simulink model "optimizer"  (R2020a)
settings: Solver=VariableStepAuto  StartTime=0.0  StopTime=10.0  RelTol=1e-3
settings Model: Creator=PIM  LastModifiedBy=PIM

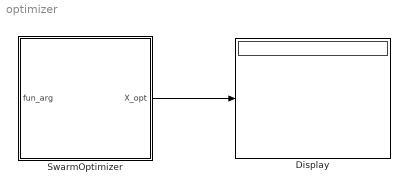
== system optimizer ==
  Display : Display
  SwarmOptimizer : MATLAB Function  TreatAsAtomicUnit=on  mask{algorithm_mask=Differential Evolution Optimizer, n_iter=100, n_particles=50, sampling_method_mask=Uniform, domain_hi=[5 5 5], domain_lo=[-5 -5 -5]}
      mask prompts: algorithm_mask "Algorithm"; n_iter "Number of iterations [float]"; n_particles "Number of particles [float]"; sampling_method_mask "Sampling method"; domain_hi "Domain Hi (array) [float]"; domain_lo "Domain Lo (array) [float]"
      mask init:
      | if strcmp(sampling_method_mask, 'Uniform')
      |     sampling_method=1;
      | elseif strcmp(sampling_method_mask, 'Cauchy')
      |     sampling_method=2;
      | elseif strcmp(sampling_method_mask, 'Normal')
      |     sampling_method=3;
      | end
      | 
      | if strcmp(algorithm_mask, 'Particle Swarm Optimizer')
      |     algorithm=1;
      | elseif strcmp(algorithm_mask, 'Differential Evolution Optimizer')
      |     algorithm=2;
      | end
  wires:
  SwarmOptimizer/1(X_opt) -> Display/1

== matlab function optimizer/SwarmOptimizer ==
  data: fun_arg input; n_particles parameter double; n_iter parameter double; domain_hi parameter double; domain_lo parameter double; sampling_method parameter double; algorithm parameter double; X_opt output size=size(domain_hi)
function X_opt=fcn(fun_arg, n_particles, n_iter, domain_hi, domain_lo, sampling_method, algorithm)
% global swarm_obj
% global topology_obj

swarm_obj=swarm;
topology_obj=topology;

%% Swarm parameters
swarm_param.n_particles=n_particles;
swarm_param.sampling_method='Uniform';
if sampling_method==1
    swarm_param.sampling_method='Uniform';
elseif sampling_method==2
    swarm_param.sampling_method='Cauchy';
elseif sampling_method==3
    swarm_param.sampling_method='Normal';
end
swarm_param.x_domain.hi=domain_hi;
swarm_param.x_domain.lo=domain_lo;

%% Algorithm parameters
alg_param.n_iter=n_iter;

alg_param.algorithm='ParticleSwarmOptimizer';
if algorithm==1
    alg_param.algorithm='ParticleSwarmOptimizer';
elseif algorithm==2
    alg_param.algorithm='DifferentialEvolutionOptimizer';
end


%% Specific configurations for Differential Evolution Algorithm
alg_param.CR    =0.9;       % crossover probability [0, 1]
alg_param.F     =0.8;       % differential weight [0, 2]

%% Specific configurations for Particle Swarm Optimizer Algorithm
alg_param.w     =0.1;       % velocity associated parameter
alg_param.c1    =0.1;       % personal best position coefficient
alg_param.c2    =0.2;       % global best position coefficient
alg_param.lr    =1;         % learning rate

X_opt=zeros(size(swarm_param.x_domain.hi));
if strcmp(alg_param.algorithm, 'DifferentialEvolutionOptimizer')
  [X_opt, y_opt]=DifferentialEvolutionOptimizer_codegen(alg_param, swarm_param, fun_arg);
end
  

end
